simulink model "PlaybackMechExplorer"  (R2024b)
settings: Solver=daessc  StartTime=0.0  StopTime=20  RelTol=0.01
undefined symbols (not defined in the file): MCU_Ts
settings Model: DataDictionary=neck_mk3.sldd  VariantConfigurationObject=Variants  Creator=upattacini  LastModifiedBy=upattacini
settings SolverCC: MaxConsecutiveMinStep=10  SolverJacobianMethodControl=FullAnalytical  DaesscMode=Robust  ZeroCrossAlgorithm=Adaptive  DecoupledContinuousIntegration=on  MinimalZcImpactIntegration=on
settings DataIOCC: SaveOutput=off  SignalLogging=off  DSMLogging=off  SaveTime=off  ReturnWorkspaceOutputs=off
settings DebuggingCC: ParameterPrecisionLossMsg=none
settings RTWCC: GPUComputeCapability=3.5
settings DiagnosticsConfigSet: SimMechanicsUnconnectedFramePorts=none
settings ExplorerConfigSet: InternalSimMechanicsExplorerSettings="<ExplorerConfiguration><canonicalview>default</canonicalview><AnimationSetting><BasePlaybackSpeed>1.0</BasePlaybackSpeed><PlaybackSpeedFactor>1.0</PlaybackSpeedFactor></AnimationSetting><TilePanel><TileInfo><Tiles Columns=\"2\" Count=\"2\" Rows=\"1\"><Column Weight=\"0.5\"/><Column Weight=\"0.5\"/><Row Weight=\"1\"/><Tile Height=\"1\" Width=\"1\" X=\"0\" Y=\"0\"/><Tile Height=\"1\" Width=\"1\" X=\"1\" Y=\"0\"/></Tiles></TileInfo><SceneInfo><SceneViewer><BGColor><R>0.60000002384185791</R><G>0.60000002384185791</G><B>0.60000002384185791</B></BGColor><Camera><DoPerspective>off</DoPerspective><Position><X>1.00000272318720818</X><Y>0.0120507962302127021</Y><Z>0.0736370887831767212</Z></Position><Center><X>2.72318720817565918e-06</X><Y>0.0120507962302127021</Y><Z>0.0736370887831767212</Z></Center><Up><X>-0</X><Y>0</Y><Z>1</Z></Up><ViewLimDist>1</ViewLimDist><YLim>0.24573583314130093</YLim><XLim>0.179173656873043957</XLim></Camera></SceneViewer><SceneViewer><BGColor><R>0.60000002384185791</R><G>0.60000002384185791</G><B>0.60000002384185791</B></BGColor><Camera><DoPerspective>off</DoPerspective><Position><X>0.00969585588153237289</X><Y>0.977383673191070335</Y><Z>0.0771038854362011</Z></Position><Center><X>0.00969585588153237289</X><Y>-0.0226163268089296585</Y><Z>0.0771038854362011</Z></Center><Up><X>0</X><Y>0</Y><Z>1</Z></Up><ViewLimDist>1</ViewLimDist><YLim>0.231031900028857928</YLim><XLim>0.168452560838758425</XLim></Camera></SceneViewer></SceneInfo></TilePanel><MechEditorPanel><Cameras/><GfxPanelCameraMap/><VideoCreator><PlaybackSpeedRatio>1.0</PlaybackSpeedRatio><FrameRate>30</FrameRate><VideoFormat>Motion JPEG AVI</VideoFormat><FrameSize>auto</FrameSize></VideoCreator></MechEditorPanel></ExplorerConfiguration>"

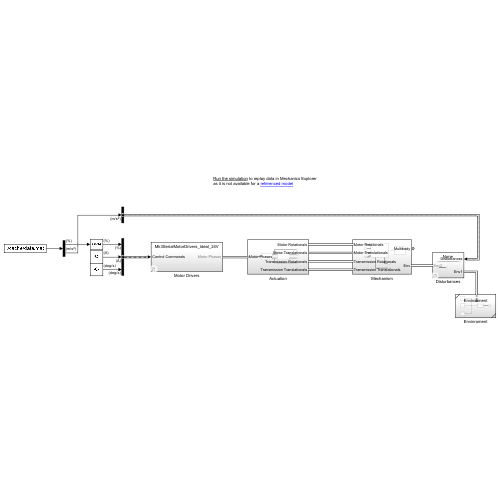
[thumbnail: Simulink's stored preview of the top-level diagram]
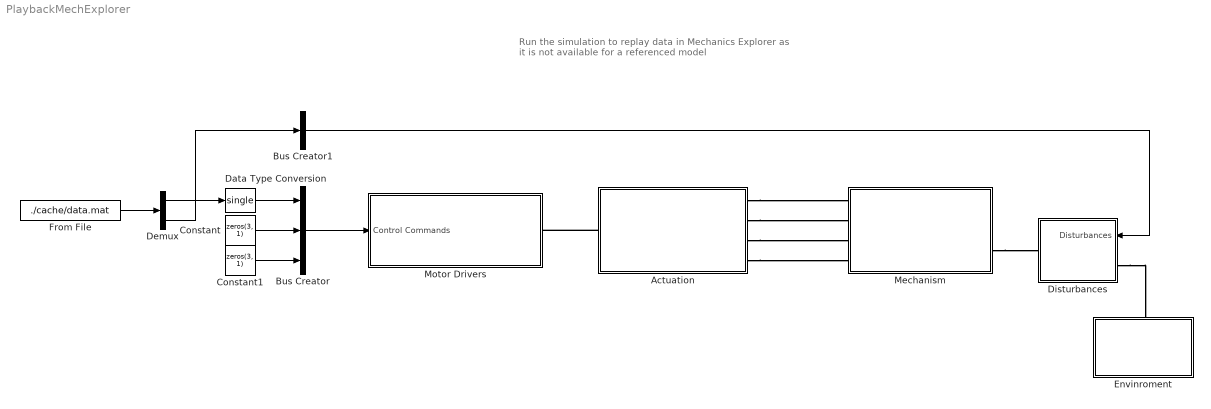
== system PlaybackMechExplorer ==
  note: Run the simulation to replay data in Mechanics Explorer
      | as it is not available for a referenced model
  Actuation : Subsystem
  Bus Creator : BusCreator  Inputs=3  OutDataTypeStr=Bus: Data_ControlCommands  NonVirtualBus=on
      settings: InheritFromInputs=off
  Bus Creator1 : BusCreator  Inputs=1  OutDataTypeStr=Bus: Data_Disturbances  NonVirtualBus=on
      settings: InheritFromInputs=off
  Constant : Constant  Value=zeros(3, 1)  OutDataTypeStr=single
  Constant1 : Constant  Value=zeros(3, 1)  OutDataTypeStr=single
  Data Type Conversion : DataTypeConversion  OutDataTypeStr=single  SaturateOnIntegerOverflow=off  RndMeth=Floor
  Demux : Demux  Outputs=2
  Disturbances : Subsystem  Variant=on  VariantControl=Disturbances
  Envinroment : Subsystem  ReferencedSubsystem=Environment
      settings: PermitHierarchicalResolution=None  PortSchema="{\"entries\":[{\"content\":{\"sides\":[{\"content\":{},\"type\":\"ConnectorPlacement.EquallySpacedRectSide\",\"uuid\":\"7683af32-0950-4752-8ae9-4c2cfa819128\"},{\"content\":{\"side\":\"RIGHT\"},\"type\":\"ConnectorPlacement.EquallySpacedRectSide\",\"uuid\":\"f63ef562-9fed-4914-8068-bf56fce23c7c\"},{\"content\":{\"connectorIds\":[\"LConn1\"],\"side\":\"TOP\"},\"type\":\"ConnectorPlacement.EquallySpacedRectSide\",\"uuid\":\"7c640675-20e8-4b81-924e-ac57cf210d7e\"}]},\"type\":\"ConnectorPlacement.EquallySpacedConnector\",\"uuid\":\"68c08bb3-7f9c-4046-9765-3cd3ae1cce69\"}],\"packageUris\":[\"http://schema.mathworks.com/mf0/Connector/R2020b\"],\"version\":\"1.0\"}"
  From File : FromFile  FileName=./cache/data.mat  SampleTime=MCU_Ts  ExtrapolationBeforeFirstDataPoint=Hold first value  InterpolationWithinTimeRange=Zero order hold  ExtrapolationAfterLastDataPoint=Hold last value
  Mechanism : Subsystem
  Motor Drivers : Subsystem  Variant=on
  wires:
  Bus Creator/1 -> Motor Drivers/1(Control Commands)
  Constant/1 -> Bus Creator/2
  Constant1/1 -> Bus Creator/3
  From File/1 -> Demux/1
  Demux/1 -> Data Type Conversion/1
  Demux/2 -> Bus Creator1/1
  Data Type Conversion/1 -> Bus Creator/1
  Bus Creator1/1 -> Disturbances/1(Disturbances)
  connections:
  Actuation/LConn1 -- Motor Drivers/RConn1
  Actuation/RConn1 -- Mechanism/LConn1
  Actuation/RConn2 -- Mechanism/LConn2
  Actuation/RConn3 -- Mechanism/LConn3
  Actuation/RConn4 -- Mechanism/LConn4
  Mechanism/RConn2 -- Disturbances/RConn1
  Disturbances/LConn1 -- Envinroment/LConn1

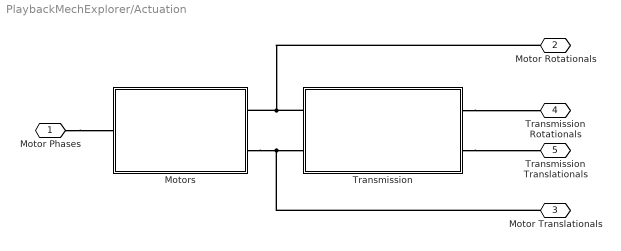
== system PlaybackMechExplorer/Actuation ==
  Motors : Subsystem  Variant=on
  Transmission : Subsystem  Variant=on
  Motor Phases : PMIOPort  Side=Left  ConnectionType=Bus: Physical_MotorPhases
  Motor Rotationals : PMIOPort  Port=2  Side=Right  ConnectionType=Bus: Physical_MotorRotationals
  Motor Translationals : PMIOPort  Port=3  Side=Right  ConnectionType=Bus: Physical_MotorTranslationals
  Transmission Rotationals : PMIOPort  Port=4  Side=Right  ConnectionType=Bus: Physical_TransmissionRotationals
  Transmission Translationals : PMIOPort  Port=5  Side=Right  ConnectionType=Bus: Physical_TransmissionTranslationals
  connections:
  Motor Phases/RConn1 -- Motors/LConn1
  Transmission/LConn1 -- Motors/RConn1 -- Motor Rotationals/RConn1
  Motors/RConn2 -- Motor Translationals/RConn1 -- Transmission/LConn2
  Transmission/RConn1 -- Transmission Rotationals/RConn1
  Transmission/RConn2 -- Transmission Translationals/RConn1

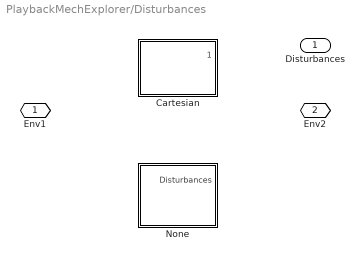
== system PlaybackMechExplorer/Disturbances ==
  Disturbances : Inport
  Cartesian : Subsystem  VariantControl=Selector_Disturbances == Types_Disturbances.Cartesian  ReferencedSubsystem=Disturbances_Cartesian
      settings: PortSchema="{\"entries\":[{\"content\":{\"sides\":[{\"content\":{\"connectorIds\":[\"In1\",\"RConn1\"]},\"type\":\"ConnectorPlacement.EquallySpacedRectSide\",\"uuid\":\"c3275bd1-611d-46ff-acae-76e496a97507\"},{\"content\":{\"connectorIds\":[\"LConn1\"],\"side\":\"RIGHT\"},\"type\":\"ConnectorPlacement.EquallySpacedRectSide\",\"uuid\":\"e38bb7c1-fa84-4003-92ff-74c07d6e999c\"},{\"content\":{\"side\":\"TOP\"},\"type\":\"ConnectorPlacement.EquallySpacedRectSide\",\"uuid\":\"ca966852-3327-4b78-bb4f-28ca7b1298e2\"}]},\"type\":\"ConnectorPlacement.EquallySpacedConnector\",\"uuid\":\"173f28ee-971a-4c77-8133-b36f3626081f\"}],\"packageUris\":[\"http://schema.mathworks.com/mf0/Connector/R2020b\"],\"version\":\"1.0\"}"
  None : Subsystem  VariantControl=Selector_Disturbances == Types_Disturbances.None
      settings: PortSchema="{\"entries\":[{\"content\":{\"sides\":[{\"content\":{\"connectorIds\":[\"LConn1\"]},\"type\":\"ConnectorPlacement.EquallySpacedRectSide\",\"uuid\":\"c3275bd1-611d-46ff-acae-76e496a97507\"},{\"content\":{\"connectorIds\":[\"In1\",\"RConn1\"],\"side\":\"RIGHT\"},\"type\":\"ConnectorPlacement.EquallySpacedRectSide\",\"uuid\":\"e38bb7c1-fa84-4003-92ff-74c07d6e999c\"},{\"content\":{\"side\":\"TOP\"},\"type\":\"ConnectorPlacement.EquallySpacedRectSide\",\"uuid\":\"ca966852-3327-4b78-bb4f-28ca7b1298e2\"}]},\"type\":\"ConnectorPlacement.EquallySpacedConnector\",\"uuid\":\"173f28ee-971a-4c77-8133-b36f3626081f\"}],\"packageUris\":[\"http://schema.mathworks.com/mf0/Connector/R2020b\"],\"version\":\"1.0\"}"
  Env1 : PMIOPort  Side=Left
  Env2 : PMIOPort  Port=2  Side=Right

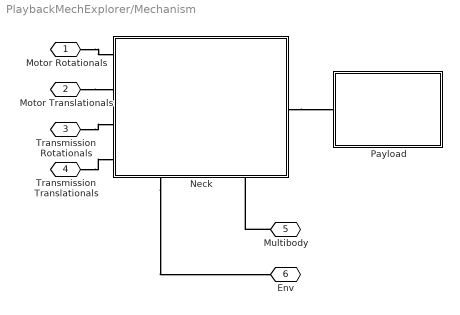
== system PlaybackMechExplorer/Mechanism ==
  Neck : Subsystem  Variant=on
      settings: PortSchema="{\"entries\":[{\"content\":{\"sides\":[{\"content\":{\"connectorIds\":[\"LConn1\",\"LConn2\",\"LConn3\",\"LConn4\"]},\"type\":\"ConnectorPlacement.EquallySpacedRectSide\",\"uuid\":\"14e513f6-3c3c-4099-84db-d86c4eb27232\"},{\"content\":{\"connectorIds\":[\"RConn1\"],\"side\":\"RIGHT\"},\"type\":\"ConnectorPlacement.EquallySpacedRectSide\",\"uuid\":\"4a464989-15a4-433b-9fcc-4a0fef6bae97\"},{\"content\":{\"side\":\"TOP\"},\"type\":\"ConnectorPlacement.EquallySpacedRectSide\",\"uuid\":\"73346d14-0c51-4cf5-8a5d-2d8850c8ad1d\"},{\"content\":{\"connectorIds\":[\"RConn2\",\"RConn3\"],\"side\":\"BOTTOM\"},\"type\":\"ConnectorPlacement.EquallySpacedRectSide\",\"uuid\":\"374f3de9-df4d-4c6c-9f7f-bd97ffef2a78\"}]},\"type\":\"ConnectorPlacement.EquallySpacedConnector\",\"uuid\":\"c700d0bc-d76f-4bb0-87b5-cee80432b7e8\"}],\"packageUris\":[\"http://schema.mathworks.com/mf0/Connector/R2020b\"],\"version\":\"1.0\"}"
  Payload : Subsystem  Variant=on
  Motor Rotationals : PMIOPort  Side=Left  ConnectionType=Bus: Physical_MotorRotationals
  Motor Translationals : PMIOPort  Port=2  Side=Left  ConnectionType=Bus: Physical_MotorTranslationals
  Transmission Rotationals : PMIOPort  Port=3  Side=Left  ConnectionType=Bus: Physical_TransmissionRotationals
  Transmission Translationals : PMIOPort  Port=4  Side=Left  ConnectionType=Bus: Physical_TransmissionTranslationals
  " Multibody" : PMIOPort  Port=5  Side=Right  ConnectionType=Bus: Physical_Multibody
  Env : PMIOPort  Port=6  Side=Right  ConnectionType=Bus: Physical_Environment
  connections:
  Neck/RConn1 -- Payload/LConn1
  " Multibody"/RConn1 -- Neck/RConn3
  Neck/RConn2 -- Env/RConn1
  Motor Rotationals/RConn1 -- Neck/LConn1
  Motor Translationals/RConn1 -- Neck/LConn2
  Transmission Rotationals/RConn1 -- Neck/LConn3
  Transmission Translationals/RConn1 -- Neck/LConn4

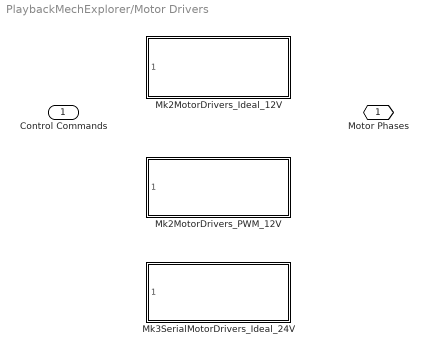
== system PlaybackMechExplorer/Motor Drivers ==
  Control Commands : Inport  OutDataTypeStr=Bus: Data_ControlCommands
  Mk2MotorDrivers_Ideal_12V : Subsystem  VariantControl=Selector_MotorDriver == Types_MotorDriver.DC_Ideal_12V  ReferencedSubsystem=Mk2MotorDrivers_Ideal
      settings: PermitHierarchicalResolution=None
  Mk2MotorDrivers_PWM_12V : Subsystem  VariantControl=Selector_MotorDriver == Types_MotorDriver.DC_PWM_12V  ReferencedSubsystem=Mk2MotorDrivers_PWM
      settings: PermitHierarchicalResolution=None
  Mk3SerialMotorDrivers_Ideal_24V : Subsystem  VariantControl=Selector_MotorDriver == Types_MotorDriver.DC_Ideal_24V  ReferencedSubsystem=Mk3SerialMotorDrivers_Ideal
      settings: PermitHierarchicalResolution=None
  Motor Phases : PMIOPort  Side=Right  ConnectionType=Bus: Physical_MotorPhases

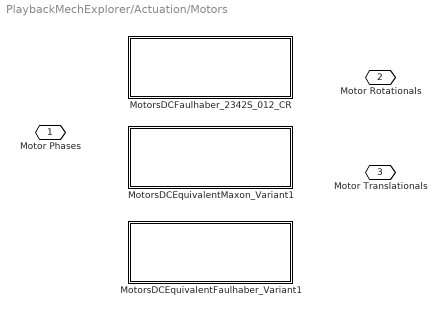
== system PlaybackMechExplorer/Actuation/Motors ==
  MotorsDCEquivalentFaulhaber_Variant1 : Subsystem  VariantControl=Selector_Motor == Types_Motor.DCEquivalent_Faulhaber_Variant1  ReferencedSubsystem=MotorsDCEquivalentFaulhaber_Variant1
      settings: PermitHierarchicalResolution=None
  MotorsDCEquivalentMaxon_Variant1 : Subsystem  VariantControl=Selector_Motor == Types_Motor.DCEquivalent_Maxon_Variant1  ReferencedSubsystem=MotorsDCEquivalentMaxon_Variant1
      settings: PermitHierarchicalResolution=None
  MotorsDCFaulhaber_2342S_012_CR : Subsystem  VariantControl=Selector_Motor == Types_Motor.DC_Faulhaber_2342S_012_CR  ReferencedSubsystem=MotorsDCFaulhaber_2342S_012_CR
      settings: PermitHierarchicalResolution=None
  Motor Phases : PMIOPort  Side=Left  ConnectionType=Bus: Physical_MotorPhases
  Motor Rotationals : PMIOPort  Port=2  Side=Right  ConnectionType=Bus: Physical_MotorRotationals
  Motor Translationals : PMIOPort  Port=3  Side=Right  ConnectionType=Bus: Physical_MotorTranslationals

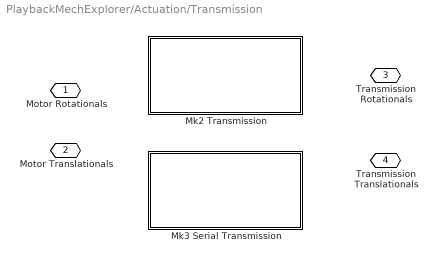
== system PlaybackMechExplorer/Actuation/Transmission ==
  Mk2 Transmission : Subsystem  VariantControl=Selector_Transmission == Types_Transmission.Mk2  ReferencedSubsystem=Mk2Transmission
      settings: PermitHierarchicalResolution=None
  Mk3 Serial Transmission : Subsystem  VariantControl=Selector_Transmission == Types_Transmission.Mk3_Serial  ReferencedSubsystem=Mk3SerialTransmission
      settings: PermitHierarchicalResolution=None
  Motor Rotationals : PMIOPort  Side=Left  ConnectionType=Bus: Physical_MotorRotationals
  Motor Translationals : PMIOPort  Port=2  Side=Left  ConnectionType=Bus: Physical_MotorTranslationals
  Transmission Rotationals : PMIOPort  Port=3  Side=Right  ConnectionType=Bus: Physical_TransmissionRotationals
  Transmission Translationals : PMIOPort  Port=4  Side=Right  ConnectionType=Bus: Physical_TransmissionTranslationals

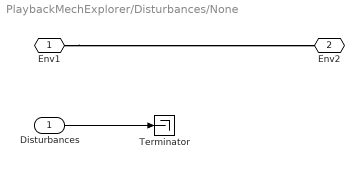
== system PlaybackMechExplorer/Disturbances/None ==
  Disturbances : Inport
  Terminator : Terminator
  Env1 : PMIOPort  Side=Left
  Env2 : PMIOPort  Port=2  Side=Right
  wires:
  Disturbances/1 -> Terminator/1
  connections:
  Env1/RConn1 -- Env2/RConn1

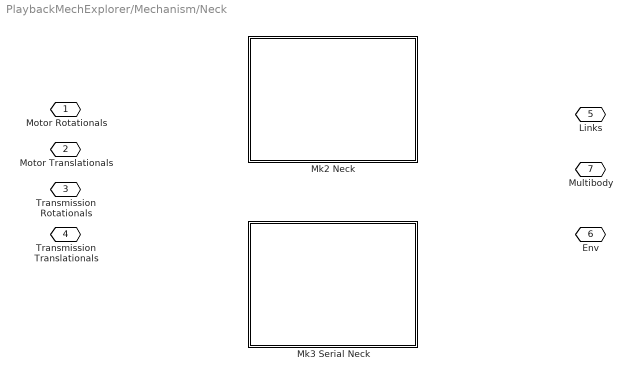
== system PlaybackMechExplorer/Mechanism/Neck ==
  Mk2 Neck : Subsystem  VariantControl=Selector_Mechanism == Types_Mechanism.Mk2  ReferencedSubsystem=Mk2NeckWrapper
      settings: PermitHierarchicalResolution=None
  Mk3 Serial Neck : Subsystem  VariantControl=Selector_Mechanism == Types_Mechanism.Mk3_Serial  ReferencedSubsystem=Mk3SerialNeckWrapper
      settings: PermitHierarchicalResolution=None
  Motor Rotationals : PMIOPort  Side=Left  ConnectionType=Bus: Physical_MotorRotationals
  Motor Translationals : PMIOPort  Port=2  Side=Left  ConnectionType=Bus: Physical_MotorTranslationals
  Transmission Rotationals : PMIOPort  Port=3  Side=Left  ConnectionType=Bus: Physical_TransmissionRotationals
  Transmission Translationals : PMIOPort  Port=4  Side=Left  ConnectionType=Bus: Physical_TransmissionTranslationals
  Links : PMIOPort  Port=5  Side=Right
  Env : PMIOPort  Port=6  Side=Right  ConnectionType=Bus: Physical_Environment
  Multibody : PMIOPort  Port=7  Side=Right  ConnectionType=Bus: Physical_Multibody

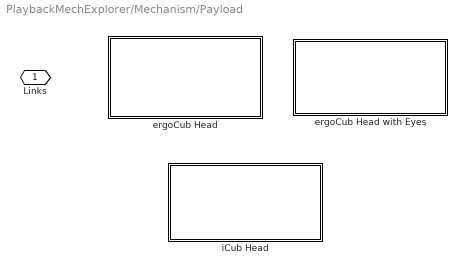
== system PlaybackMechExplorer/Mechanism/Payload ==
  ergoCub Head : Subsystem  VariantControl=Selector_Payload == Types_Payload.ergoCubHead  ReferencedSubsystem=ergoCubHeadWrapper
      settings: PermitHierarchicalResolution=None
  ergoCub Head with Eyes : Subsystem  VariantControl=Selector_Payload == Types_Payload.ergoCubHeadWithEyes  ReferencedSubsystem=ergoCubHeadWithEyesWrapper
      settings: PermitHierarchicalResolution=None
  iCub Head : Subsystem  VariantControl=Selector_Payload == Types_Payload.iCubHead  ReferencedSubsystem=iCubHeadWrapper
  Links : PMIOPort  Side=Left
